simulink library "SunTorqueA"  (R2014b)
settings: Solver=ode45  StartTime=0.0  StopTime=10.0  RelTol=1e-3
libraries: LeverArm x1, SunForce_sat x1, CrossProd x1
settings Model: Creator=Hp  LastModifiedBy=Hp

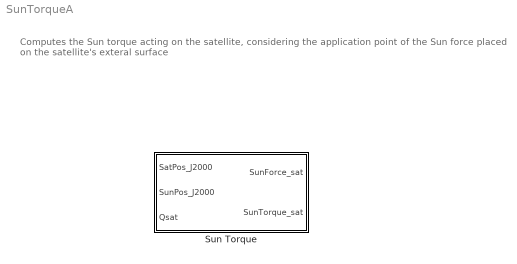
== system SunTorqueA ==
  note: Computes the Sun torque acting on the satellite,
      | considering the application point of the Sun force
      | placed on the satellite's exteral surface
  Sun Torque : Subsystem

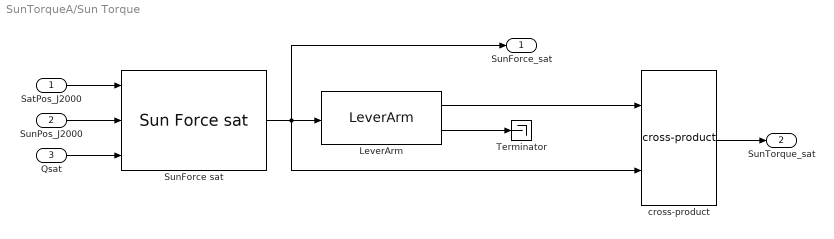
== system SunTorqueA/Sun Torque ==
  SatPos_J2000 : Inport
  SunPos_J2000 : Inport  Port=2
  Qsat : Inport  Port=3
  LeverArm : LeverArm/LeverArm
  SunForce sat : SunForce_sat/Sun Force sat
  Terminator : Terminator
  cross-product : CrossProd/cross-product
  SunForce_sat : Outport
  SunTorque_sat : Outport  Port=2
  wires:
  LeverArm/1 -> cross-product/1
  SatPos_J2000/1 -> SunForce sat/1
  Qsat/1 -> SunForce sat/3
  cross-product/1 -> SunTorque_sat/1
  SunForce sat/1 -> SunForce_sat/1, cross-product/2, LeverArm/1
  SunPos_J2000/1 -> SunForce sat/2
  LeverArm/2 -> Terminator/1
